simulink model "sgMdl_IO3xx_SENT_serialMessagesSPC"  (R2024b)
settings: Solver=FixedStepAuto  StartTime=0.0  StopTime=inf  RelTol=1e-3  EnableMultiTasking=on
undefined symbols (not defined in the file): Pull, pull, up
libraries: simulink x4, hdlsllib x2, speedgoatlib_fpga_sent x2, speedgoatlib_fpga x1
Description:
  | SENT - Serial Messages SPC
settings Model: ModifiedByFormat=Speedgoat  SimulationMode=external  ExtModeTrigDuration=100000  Creator=Speedgoat  LastModifiedBy=Speedgoat
settings SolverCC: ConcurrentTasks=on  AlgebraicLoopSolver=TrustRegion  PositivePriorityOrder=on  AutoInsertRateTranBlk=on  InsertRTBMode=Never (minimum delay)
settings DataIOCC: SaveFormat=StructureWithTime
settings OptimizationCC: BlockReduction=off  OptimizeBlockIOStorage=off  BufferReuse=off
settings DebuggingCC: UnderspecifiedInitializationDetection=Classic  MergeDetectMultiDrivingBlocksExec=none  TasksWithSamePriorityMsg=none
settings HardwareCC: ProdBitPerLong=64  ProdLongLongMode=on  ProdHWDeviceType=Intel->x86-64 (Linux 64)
settings ModelReferenceCC: EnableRefExpFcnMdlSchedulingChecks=on  PropagateSignalLabelsOutOfModel=off
settings RTWCC: Description=Speedgoat Real-Time Target Machine  SystemTargetFile=speedgoat.tlc  TLCOptions=-axpcCPUClockPoll=0  TemplateMakefile=slrealtime_default_tmf  Toolchain=Simulink Real-Time Toolchain  BuildConfiguration=Faster Runs  TargetLang=C++  GPUComputeCapability=3.5  DLArmComputeVersion=19.05
settings SimulinkRealTimeTargetCC: SubcomponentCodeInterfacePackaging=Reusable function  MATLABClassNameForMDSCustomization=Simulink.SoftwareTarget.GRTCustomization  InstructionSetFMA=off  LogToMDFFile=off  SLRTFileLogMaxRuns=10
settings ConfigComp: CovBoundaryAbsTol=1.0e-5

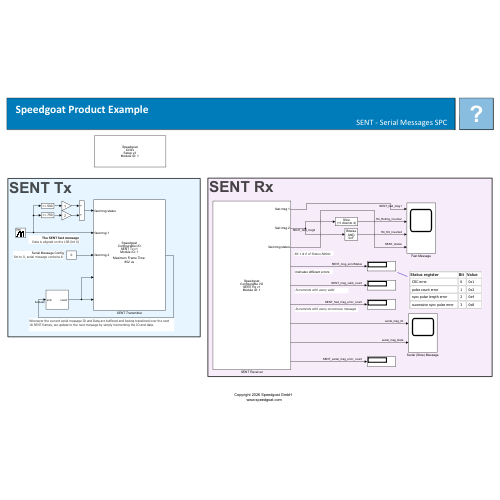
[thumbnail: Simulink's stored preview of the top-level diagram]
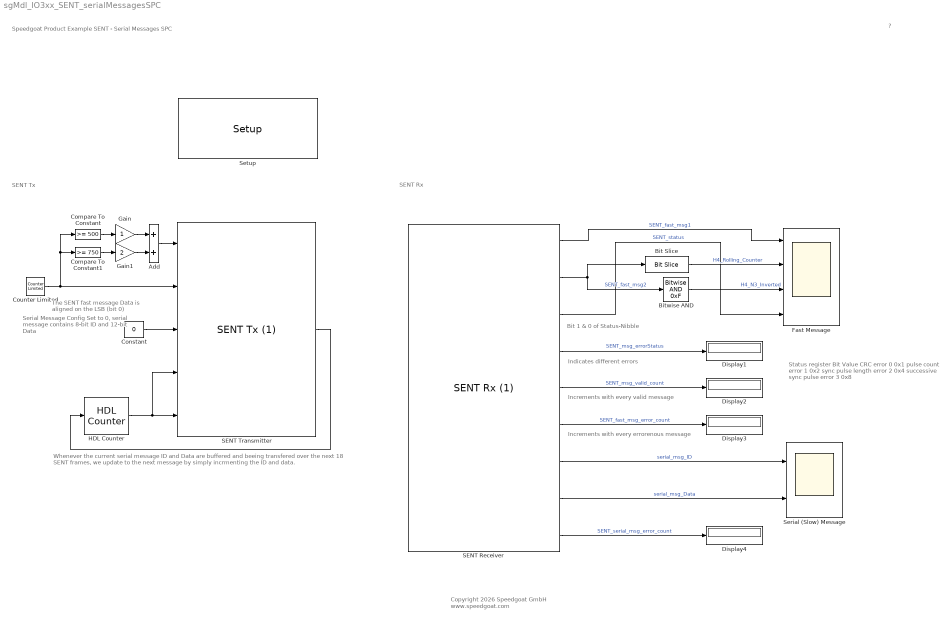
== system sgMdl_IO3xx_SENT_serialMessagesSPC ==
  note: SENT Tx
  note: The SENT fast message
      | Data is aligned on the LSB (bit 0)
  note: Increments with every valid message
  note: SENT Rx
  note: Increments with every errorenous message
  note: Indicates different errors
  note: Status register
      | Bit
      | Value
      |
      | CRC error
      | 0
      | 0x1
      |
      | pulse count error
      | 1
      | 0x2
      |
      | sync pulse length error
      | 2
      | 0x4
      |
      | successive sync pulse error
      | 3
      | 0x8
  note: Bit 1 & 0 of Status-Nibble
  note: Serial Message Config
      | Set to 0, serial message contains 8-bit ID and 12-bit Data
  note: Whenever the current serial message ID and Data are buffered and beeing transfered over the next 18 SENT frames, we update to the next message by simply incrmenting the ID and data.
  note: Speedgoat Product Example
      | SENT - Serial Messages SPC
  note: ?
  note: Copyright 2026 Speedgoat GmbH
      |  www.speedgoat.com
  Add : Sum  OutDataTypeStr=Inherit: Inherit via back propagation
  Bit Slice : hdlsllib/Logic and Bit Operations/Bit Slice  lidx=11  ridx=4
  Bitwise AND : simulink/Logic and Bit Operations/Bitwise Operator  logicop=AND  UseBitMask=on  BitMask=0xF  BitMaskRealWorld=Stored Integer
      settings: LibrarySourceBlock=|
      | simulink/Quick Insert/Logic and Bit
      | Operations/Bitwise AND
  Compare To Constant : simulink/Logic and Bit Operations/Compare To Constant  relop=>=  const=500  OutDataTypeStr=uint8
  Compare To Constant1 : simulink/Logic and Bit Operations/Compare To Constant  relop=>=  const=750  OutDataTypeStr=uint8
  Constant : Constant  Value=0  OutDataTypeStr=Inherit: Inherit via back propagation  SampleTime=-1
  Counter Limited : simulink/Sources/Counter Limited  uplimit=999  tsamp=1e-3
  Display{1..4} (4 alike) : Display
  Fast Message : Scope  NumInputPorts=4
  Gain : Gain  OutDataTypeStr=Inherit: Inherit via back propagation
  Gain1 : Gain  Gain=2  OutDataTypeStr=Inherit: Inherit via back propagation
  HDL Counter : hdlsllib/Sources/HDL Counter  CountType=Free running  CountInit=0  CountStep=1  CountMax=25  CountFromType=Initial value  CountFrom=0  CountResetPort=off  CountLoadPort=off  CountEnbPort=on  CountDirPort=off  CountHitOutputPort=off  CountDataType=Unsigned  CountWordLen=16  CountFracLen=0  CountSampTime=1
  SENT Receiver : speedgoatlib_fpga_sent/SENT Rx (1)  id=1  chan=1  ts=-1  tick_length=[3e-6]  spc_mode=Synchronous Transmission  data_format=Secure sensor with 12-bit fast channel 1 and secure sensor information on fast channel 2 (H.4)  nbr_nibbles=2  enable_pause=on  enable_raw_mode=on  legacy_crc=Recommended CRC  status_in_crc=on  useDefaultCrcPolynom=on  crcPolynom=0b1101  crcInit=0b0011  enable_enhanced_serial_messages=on  showStatus=on  showErrState=on  showValidCntr=on  showErrorCntr=on
      settings: SourceProductName=SENT
  SENT Transmitter : speedgoatlib_fpga_sent/SENT Tx (1)  id=1  chan=1  ts=-1  tick_length=[3e-6]  spc_mode=Synchronous Transmission  data_format=Secure sensor with 12-bit fast channel 1 and secure sensor information on fast channel 2 (H.4)  nbr_nibbles=2  frameTriggerEn=on  invertedSENT=off  enable_pause=off  variable_pause_length=off  pause_length=[50]  enable_enhanced_serial_messages=on  legacy_crc=Recommended CRC  status_in_crc=on  useDefaultCrcPolynom=on  crcPolynom=0b1101  crcInit=0b0011
      settings: SourceProductName=SENT
  Serial (Slow) Message : Scope  NumInputPorts=2
  Setup : speedgoatlib_fpga/Setup/Setup  board=Please select...  id=1  pciSlot=-1  device_id=1  bitstreamFilePath=C:\Work\SVN\Speedgoatlib\trunk\product_examples\IO3xx_SENT\IO3xx_SENT_helper\  bitstreamFile=Please select...  fpgaFreq=75e6  enableDma=off  rearEnb_1=off  rearIO_1=None  rearEnb_2=off  rearIO_2=None  ProgSpiFlash=off  ProgBPIFlash=off  useFpgaDmaController=off  dmaTrigDropdown=Model Step  dmaTrigSelect=0  dmaStopOnOverload=on  dmaModeSequential=on  dmaModeParallel=off  PullRPort15=pull-up 3.3V  PullRPort31=pull-up 3.3V  PullRPort47=pull-up 3.3V  PullRPort63=pull-up 3.3V  diffLineTermination_1=on  diffLineTermination_2=on  diffLineTermination_3=on  diffLineTermination_4=on  diffLineTermination_5=on  diffLineTermination_6=on  diffLineTermination_7=on  diffLineTermination_8=on  diffLineTermination_9=on  diffLineTermination_10=on  diffLineTermination_11=on  diffLineTermination_12=on  diffLineTermination_13=on  diffLineTermination_14=on  diffLineTermination_15=on  diffLineTermination_16=on  diffLineTermination_17=on  diffLineTermination_18=on  diffLineTermination_19=on  diffLineTermination_20=on  diffLineTermination_21=on  diffLineTermination_22=on  diffLineTermination_23=on  diffLineTermination_24=on  diffLineTermination_25=on  diffLineTermination_26=on  diffLineTermination_27=on  diffLineTermination_28=on  diffLineTermination_29=on  diffLineTermination_30=on  diffLineTermination_31=on  diffLineTermination_32=on  ioVoltageDropDown1=3.3V  pullResistorDropDown1_1=Pull-up  pullResistorDropDown1_2=Pull-up  pullResistorDropDown1_3=Pull-up  pullResistorDropDown1_4=Pull-up  pullResistorDropDown1_5=Pull-up  pullResistorDropDown1_6=Pull-up  pullResistorDropDown1_7=Pull-up  pullResistorDropDown1_8=Pull-up  ttlIsImplementedCheckBox1=off  pullResistorDropDown2=Pull-up  ioVoltageDropDown2=3.3V  ttlIsImplementedCheckBox2=off  pullResistorDropDown3=Pull-up  ioVoltageDropDown3=3.3V  ttlIsImplementedCheckBox3=off  pullResistorDropDown4=Pull-up  ioVoltageDropDown4=3.3V  ttlIsImplementedCheckBox4=off  pullResistorDropDown5=Pull-up  ioVoltageDropDown5=3.3V  ttlIsImplementedCheckBox5=off  pullResistorDropDown6=Pull-up  ioVoltageDropDown6=3.3V  ttlIsImplementedCheckBox6=off  pullResistorDropDown7=Pull-up  ioVoltageDropDown7=3.3V  ttlIsImplementedCheckBox7=off  pullResistorDropDown8=Pull-up  ioVoltageDropDown8=3.3V  ttlIsImplementedCheckBox8=off  terminationCheckBox1=off  terminationCheckBox2=off  terminationCheckBox3=off  terminationCheckBox4=off  diffIsImplementedCheckBox1=off  terminationCheckBox5=off  terminationCheckBox6=off  terminationCheckBox7=off  terminationCheckBox8=off  diffIsImplementedCheckBox2=off  terminationCheckBox9=off  terminationCheckBox10=off  terminationCheckBox11=off  terminationCheckBox12=off  diffIsImplementedCheckBox3=off  terminationCheckBox13=off  terminationCheckBox14=off  terminationCheckBox15=off  terminationCheckBox16=off  diffIsImplementedCheckBox4=off  terminationCheckBox17=off  terminationCheckBox18=off  terminationCheckBox19=off  terminationCheckBox20=off  diffIsImplementedCheckBox5=off  terminationCheckBox21=off  terminationCheckBox22=off  terminationCheckBox23=off  terminationCheckBox24=off  diffIsImplementedCheckBox6=off  terminationCheckBox25=off  terminationCheckBox26=off  terminationCheckBox27=off  terminationCheckBox28=off  diffIsImplementedCheckBox7=off  terminationCheckBox29=off  terminationCheckBox30=off  terminationCheckBox31=off  terminationCheckBox32=off  diffIsImplementedCheckBox8=off  PullRPort0_1=pull-up  VioPort0_1=3.3V  PullRPort1_1=pull-up  VioPort1_1=3.3V  PullRPort2_1=pull-up  VioPort2_1=3.3V  PullRPort3_1=pull-up  VioPort3_1=3.3V  PullRPort4_1=pull-up  VioPort4_1=3.3V  PullRPort5_1=pull-up  VioPort5_1=3.3V  PullRPort6_1=pull-up  VioPort6_1=3.3V  diffLineTermination_rear1_1=on  diffLineTermination_rear1_2=on  diffLineTermination_rear1_3=on  diffLineTermination_rear1_4=on  diffLineTermination_rear1_5=on  diffLineTermination_rear1_6=on  diffLineTermination_rear1_7=on  diffLineTermination_rear1_8=on  PullRPort0_2=pull-up  VioPort0_2=3.3V  PullRPort1_2=pull-up  VioPort1_2=3.3V  PullRPort2_2=pull-up  VioPort2_2=3.3V  PullRPort3_2=pull-up  VioPort3_2=3.3V  PullRPort4_2=pull-up  VioPort4_2=3.3V  PullRPort5_2=pull-up  VioPort5_2=3.3V  PullRPort6_2=pull-up  VioPort6_2=3.3V  diffLineTermination_rear2_1=on  diffLineTermination_rear2_2=on  diffLineTermination_rear2_3=on  diffLineTermination_rear2_4=on  diffLineTermination_rear2_5=on  diffLineTermination_rear2_6=on  diffLineTermination_rear2_7=on  diffLineTermination_rear2_8=on
      settings: SourceProductName=IO3xx
  wires:
  SENT Receiver/3 -> Fast Message/4  "SENT_status"
  SENT Receiver/1 -> Fast Message/1  "SENT_fast_msg1"
  Add/1 -> SENT Transmitter/1
  Counter Limited/1 -> Compare To Constant/1, Compare To Constant1/1, SENT Transmitter/2
  SENT Receiver/4 -> Display1/1  "SENT_msg_errorStatus"
  Compare To Constant1/1 -> Gain1/1
  SENT Receiver/5 -> Display2/1  "SENT_msg_valid_count"
  Gain/1 -> Add/1
  SENT Receiver/6 -> Display3/1  "SENT_fast_msg_error_count"
  Gain1/1 -> Add/2
  Compare To Constant/1 -> Gain/1
  Constant/1 -> SENT Transmitter/3
  HDL Counter/1 -> SENT Transmitter/4, SENT Transmitter/5
  SENT Transmitter/1 -> HDL Counter/1
  Bit Slice/1 -> Fast Message/2  "H4_Rolling_Counter"
  Bitwise AND/1 -> Fast Message/3  "H4_N3_Inverted"
  SENT Receiver/2 -> Bitwise AND/1, Bit Slice/1  "SENT_fast_msg2"
  SENT Receiver/7 -> Serial (Slow) Message/1  "serial_msg_ID"
  SENT Receiver/8 -> Serial (Slow) Message/2  "serial_msg_Data"
  SENT Receiver/9 -> Display4/1  "SENT_serial_msg_error_count"
